simulink library "RGPbasedSetpointControl"  (R2019b)
settings: Solver=VariableStepAuto  StartTime=0.0  StopTime=10.0  RelTol=1e-3
undefined symbols (not defined in the file or in its folder): basisCovMat, basisVector, hyperParameters, meanFcnProperties, meanFcnVector, noiseVariance, postVarCtrlGain, predMeanCtrlGain
libraries: simulink x1, RGP_ctrl x1, RGP_objF x1, RGP_regression x1, flowSpeedCtrl x1, processRawData x1, makeOcB_cl x1
settings Model: Creator=Ayaz  LastModifiedBy=Ayaz

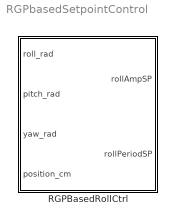
== system RGPbasedSetpointControl ==
  RGPBasedRollCtrl : Subsystem  mask{FilterWindowSize=20, vRated=20, xBasis=basisVector, meanFcnProp=meanFcnProperties, meanFcnVec=meanFcnVector, hyperParams=hyperParameters, basisCovMat=basisCovMat, noiseVar=noiseVariance, predMeanGain=predMeanCtrlGain, postVarGain=2^postVarCtrlGain, initRollAmpDeg=0, initRollPeriodSec=20, ctrlTriggerInt=3}
      mask prompts: FilterWindowSize "Filter window size"; vRated "Turbine rated speed [cm/s]"; xBasis "Basis vector"; meanFcnProp "Mean function properties"; meanFcnVec "Mean function vector"; hyperParams "Covariance hyperparameters"; basisCovMat "Basis vectors covariance matrix"; noiseVar "Noise variance"; predMeanGain "Prediction mean gain"; postVarGain "Posterior variance gain"; initRollAmpDeg "Initial roll amplitude [deg]"; initRollPeriodSec "Initial roll period [sec]"; ctrlTriggerInt "Control trigger intervals"
      mask TypeOptions FilterWindowSize: processRawData/FilterWindowSize
      mask TypeOptions vRated: RGP_objF/vRated
      mask TypeOptions xBasis: RGP_regression/xBasis | RGPBasedRollCtrl/xBasis
      mask TypeOptions meanFcnProp: RGP_regression/meanFcnProp
      mask TypeOptions meanFcnVec: RGP_regression/meanFcnVec
      mask TypeOptions hyperParams: RGP_regression/hyperParams
      mask TypeOptions basisCovMat: RGP_regression/basisCovMat
      mask TypeOptions noiseVar: RGP_regression/noiseVar
      mask TypeOptions predMeanGain: RGPBasedRollCtrl/predMeanGain
      mask TypeOptions postVarGain: RGPBasedRollCtrl/postVarGain
      mask TypeOptions initRollAmpDeg: RGPBasedRollCtrl/initRollAmpDeg
      mask TypeOptions initRollPeriodSec: RGPBasedRollCtrl/initRollPeriodSec
      mask TypeOptions ctrlTriggerInt: Constant2/Value
      mask DialogControl ParameterGroupVar Prompt: Data filtering
      mask DialogControl Container3 Prompt: RGP regression
      mask DialogControl Container4 Prompt: RGP control

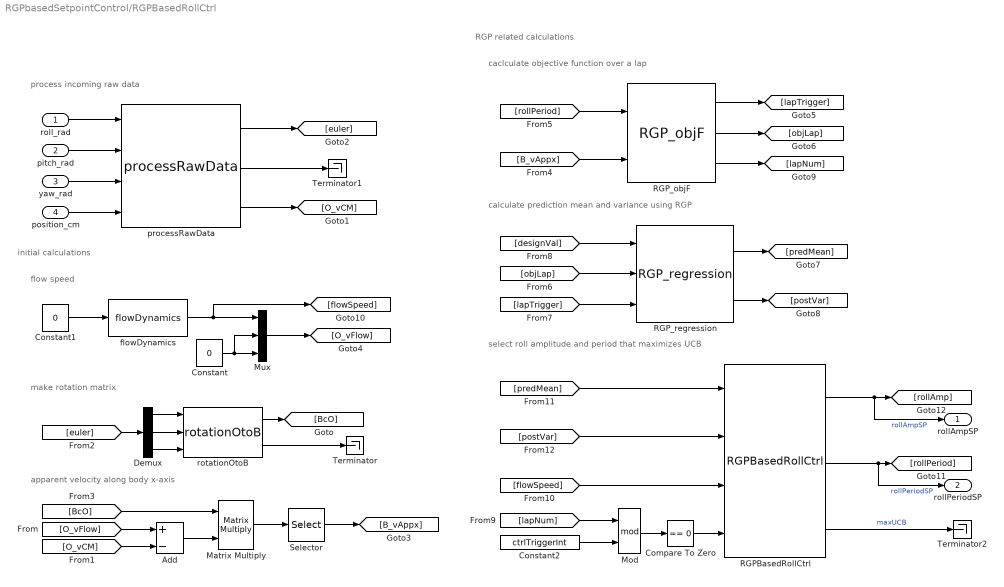
== system RGPbasedSetpointControl/RGPBasedRollCtrl ==
  note: process incoming raw data
  note: RGP related calculations
  note: select roll amplitude and period that maximizes UCB
  note: calculate prediction mean and variance using RGP
  note: caclculate objective function over a lap
  note: initial calculations
  note: apparent velocity along body x-axis
  note: flow speed
  note: make rotation matrix
  roll_rad : Inport
  pitch_rad : Inport  Port=2
  yaw_rad : Inport  Port=3
  position_cm : Inport  Port=4
  Add : Sum  Inputs=+-
  Compare To Zero : simulink/Logic and Bit Operations/Compare To Zero  relop===  OutDataTypeStr=boolean
  Constant : Constant  Value=0
  Constant1 : Constant  Value=0
  Constant2 : Constant  Value=ctrlTriggerInt
  Demux : Demux  Outputs=3
  Matrix Multiply : Product  Multiplication=Matrix(*)
  Mod : Math  Operator=mod  SaturateOnIntegerOverflow=on
  Mux : Mux  Inputs=3
  RGPBasedRollCtrl : RGP_ctrl/RGPBasedRollCtrl  predMeanGain=predMeanGain  postVarGain=postVarGain  xBasis=xBasis  initRollAmpDeg=initRollAmpDeg  initRollPeriodSec=initRollPeriodSec
  RGP_objF : RGP_objF/RGP_objF  vRated=vRated
  RGP_regression : RGP_regression/RGP_regression  xBasis=xBasis  meanFcnProp=meanFcnProp  meanFcnVec=meanFcnVec  hyperParams=hyperParams  basisCovMat=basisCovMat  noiseVar=noiseVar
  Selector : Selector  InputPortWidth=3  IndexOptions=Index vector (dialog)  Indices=1  OutputSizes=1
  Terminator : Terminator
  Terminator1 : Terminator
  Terminator2 : Terminator
  flowDynamics : flowSpeedCtrl/flowDynamics  SystemSampleTime=-1  Latency=0  AutoFrameSizeCalculation=off
  processRawData : processRawData/processRawData  FilterWindowSize=FilterWindowSize
  rotationOtoB : makeOcB_cl/rotationOtoB  SystemSampleTime=-1  Latency=0  AutoFrameSizeCalculation=off
  rollAmpSP : Outport
  rollPeriodSP : Outport  Port=2
  wires:
  RGP_regression/2 -> [postVar]
  yaw_rad/1 -> processRawData/3
  Constant/1 -> Mux/2, Mux/3
  [rollPeriod] -> RGP_objF/1
  RGP_regression/1 -> [predMean]
  [O_vCM] -> Add/2
  [euler] -> Demux/1
  Demux/3 -> rotationOtoB/3
  rotationOtoB/2 -> Terminator/1
  flowDynamics/1 -> [flowSpeed], Mux/1
  RGP_objF/2 -> [objLap]
  RGPBasedRollCtrl/3 -> Terminator2/1  "maxUCB"
  Demux/1 -> rotationOtoB/1
  processRawData/1 -> [euler]
  [O_vFlow] -> Add/1
  RGP_objF/3 -> [lapNum]
  Demux/2 -> rotationOtoB/2
  [designVal] -> RGP_regression/1
  Mux/1 -> [O_vFlow]
  [lapTrigger] -> RGP_regression/3
  processRawData/3 -> [O_vCM]
  processRawData/2 -> Terminator1/1
  [objLap] -> RGP_regression/2
  Add/1 -> Matrix Multiply/2
  position_cm/1 -> processRawData/4
  RGPBasedRollCtrl/1 -> [rollAmp], rollAmpSP/1  "rollAmpSP"
  [BcO] -> Matrix Multiply/1
  Matrix Multiply/1 -> Selector/1
  Compare To Zero/1 -> RGPBasedRollCtrl/4
  Constant1/1 -> flowDynamics/1
  Mod/1 -> Compare To Zero/1
  rotationOtoB/1 -> [BcO]
  roll_rad/1 -> processRawData/1
  Selector/1 -> [B_vAppx]
  [predMean] -> RGPBasedRollCtrl/1
  [lapNum] -> Mod/1
  [B_vAppx] -> RGP_objF/2
  Constant2/1 -> Mod/2
  RGP_objF/1 -> [lapTrigger]
  [flowSpeed] -> RGPBasedRollCtrl/3
  [postVar] -> RGPBasedRollCtrl/2
  RGPBasedRollCtrl/2 -> rollPeriodSP/1, [rollPeriod]  "rollPeriodSP"
  pitch_rad/1 -> processRawData/2
